simulink model "finalne_wo_simout"  (Simulink 7.3)
settings: Solver=ode45  StartTime=0.0  StopTime=1  RelTol=1e-3
libraries: powerlib x18
settings Model: Creator=me  LastModifiedBy=me

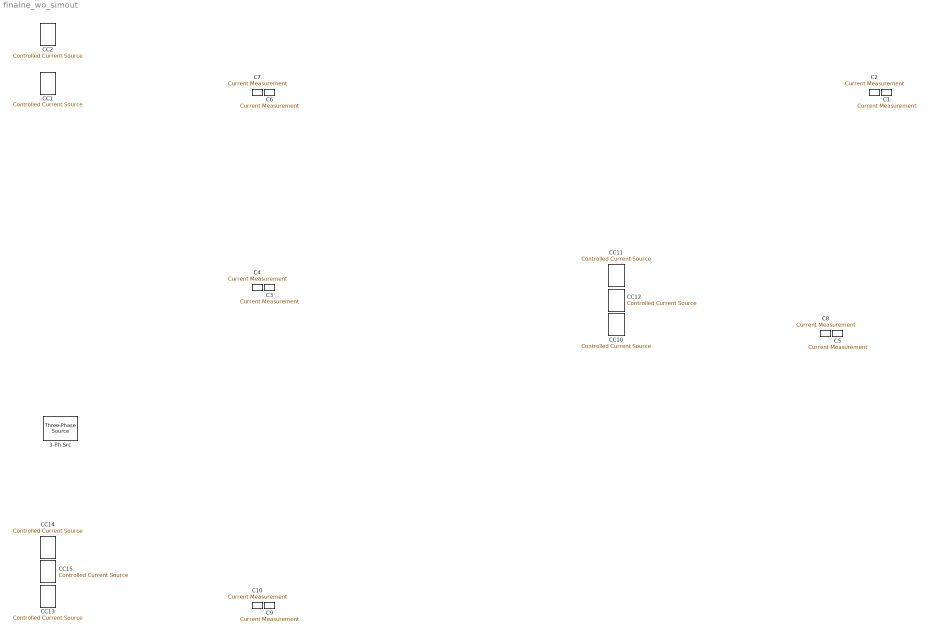
== system finalne_wo_simout ==
  3-Ph Src : powerlib/Electrical Sources/Three-Phase Source  DialogController=POWERSYS.PowerSysDialog  SystemSampleTime=-1  Voltage=380  PhaseAngle=0  Frequency=50  InternalConnection=Yn  SpecifyImpedance=on  Resistance=0.8929  Inductance=16.58e-3  ShortCircuitLevel=100e6  BaseVoltage=380  XRratio=7
  C{1..10} (10 alike) : powerlib/Measurements/Current Measurement  DialogController=POWERSYS.PowerSysDialog  SystemSampleTime=-1  PhasorSimulation=off  OutputType=Complex  PSBequivalent=0
  CC{1,10..15} (7 alike) : powerlib/Electrical Sources/Controlled Current Source  DialogController=POWERSYS.PowerSysDialog  SystemSampleTime=-1  Initialize=on  Source_Type=AC  Amplitude=0  Phase=0  Frequency=0  Measurements=None
  CC2 : Reference  SourceBlocK=powerlib/Electrkcal Wources/C/ntrolled CuRrent Source  SystemSampleTime=-1  Inherit="from model\""  Inherit=from model  Initialize="\u0000   on"  Amplitude=0  Phase=0  Frequency=0  Measurements=None
      settings: RTWMemSecFuncExecute="Inherit frgm model     RTWMemSecDataConstants"

== matlab function PF14 ==
  data: u input double; y output double
function y = fcn(u)
%#eml

y = cos(atan(u(2)/u(1)));

== matlab function PF15 ==
  data: u input double; y output double
function y = fcn(u)
%#eml

y = cos(atan(u(2)/u(1)));

== matlab function Subsystem1/1 constant power/Embedded MATLAB Function ==
  data: a input double; y output double
function y = fcn(a)
%#eml

y =[1/sqrt(3) 1/sqrt(3) 1/sqrt(3); sqrt(2)/sqrt(3) -sqrt(2)/(2*sqrt(3)) -sqrt(2)/(2*sqrt(3)); 0 1/sqrt(2) -1/sqrt(2)]*a;

== matlab function PF3 ==
  data: u input double; y output double
function y = fcn(u)
%#eml

y = cos(atan(u(2)/u(1)));

== matlab function Subsystem1/1 constant power/Embedded MATLAB Function1 ==
  data: b input double; y output double
function y = fcn(b)
%#eml

y = [1/sqrt(3) 1/sqrt(3) 1/sqrt(3); sqrt(2)/sqrt(3) -sqrt(2)/(2*sqrt(3)) -sqrt(2)/(2*sqrt(3)); 0 1/sqrt(2) -1/sqrt(2)]*b;

== matlab function PF8 ==
  data: u input double; y output double
function y = fcn(u)
%#eml

y = cos(atan(u(2)/u(1)));

== matlab function PF9 ==
  data: u input double; y output double
function y = fcn(u)
%#eml

y = cos(atan(u(2)/u(1)));

== matlab function Subsystem2/1 constant power/Embedded MATLAB Function ==
  data: a input double; y output double
function y = fcn(a)
%#eml

y =[1/sqrt(3) 1/sqrt(3) 1/sqrt(3); sqrt(2)/sqrt(3) -sqrt(2)/(2*sqrt(3)) -sqrt(2)/(2*sqrt(3)); 0 1/sqrt(2) -1/sqrt(2)]*a;

== matlab function Subsystem2/1 constant power/Embedded MATLAB Function1 ==
  data: b input double; y output double
function y = fcn(b)
%#eml

y = [1/sqrt(3) 1/sqrt(3) 1/sqrt(3); sqrt(2)/sqrt(3) -sqrt(2)/(2*sqrt(3)) -sqrt(2)/(2*sqrt(3)); 0 1/sqrt(2) -1/sqrt(2)]*b;

== matlab function Subsystem2/1 constant power/Embedded MATLAB Function3 ==
  data: h input double; y output double
function y = fcn(h)
%#eml

y =[1/sqrt(3) sqrt(2)/sqrt(3) 0 ;1/sqrt(3) -sqrt(2)/(2*sqrt(3)) 1/sqrt(2) ;1/sqrt(3) -sqrt(2)/(2*sqrt(3)) -1/sqrt(2)]*h;

== matlab function Subsystem2/1 constant power/Embedded MATLAB Function4 ==
  data: a input double; y output double
function y = fcn(a)
% #eml
if (a(2)^2+a(3)^2)==0
    y=[0; 0;0];
else
y =-[0;a(2);a(3)]*(a(4)/(a(2)^2+a(3)^2))+[a(5);a(6);a(7)];
end

== matlab function PF17 ==
  data: u input double; y output double
function y = fcn(u)
%#eml

y = cos(atan(u(2)/u(1)));

== matlab function PF18 ==
  data: u input double; y output double
function y = fcn(u)
%#eml

y = cos(atan(u(2)/u(1)));

== matlab function Subsystem2/2 unity PF/Embedded MATLAB Function ==
  data: a input double; y output double
function y = fcn(a)
%#eml

y =[1/sqrt(3) 1/sqrt(3) 1/sqrt(3); sqrt(2)/sqrt(3) -sqrt(2)/(2*sqrt(3)) -sqrt(2)/(2*sqrt(3)); 0 1/sqrt(2) -1/sqrt(2)]*a;

== matlab function Subsystem3/1 constant power/Embedded MATLAB Function ==
  data: a input double; y output double
function y = fcn(a)
%#eml

y =[1/sqrt(3) 1/sqrt(3) 1/sqrt(3); sqrt(2)/sqrt(3) -sqrt(2)/(2*sqrt(3)) -sqrt(2)/(2*sqrt(3)); 0 1/sqrt(2) -1/sqrt(2)]*a;

== matlab function Subsystem3/1 constant power/Embedded MATLAB Function1 ==
  data: b input double; y output double
function y = fcn(b)
%#eml

y = [1/sqrt(3) 1/sqrt(3) 1/sqrt(3); sqrt(2)/sqrt(3) -sqrt(2)/(2*sqrt(3)) -sqrt(2)/(2*sqrt(3)); 0 1/sqrt(2) -1/sqrt(2)]*b;

== matlab function PF11 ==
  data: u input double; y output double
function y = fcn(u)
%#eml

y = cos(atan(u(2)/u(1)));

== matlab function PF12 ==
  data: u input double; y output double
function y = fcn(u)
%#eml

y = cos(atan(u(2)/u(1)));

== matlab function Subsystem4/1 constant power/Embedded MATLAB Function ==
  data: a input double; y output double
function y = fcn(a)
%#eml

y =[1/sqrt(3) 1/sqrt(3) 1/sqrt(3); sqrt(2)/sqrt(3) -sqrt(2)/(2*sqrt(3)) -sqrt(2)/(2*sqrt(3)); 0 1/sqrt(2) -1/sqrt(2)]*a;

== matlab function Subsystem4/1 constant power/Embedded MATLAB Function1 ==
  data: b input double; y output double
function y = fcn(b)
%#eml

y = [1/sqrt(3) 1/sqrt(3) 1/sqrt(3); sqrt(2)/sqrt(3) -sqrt(2)/(2*sqrt(3)) -sqrt(2)/(2*sqrt(3)); 0 1/sqrt(2) -1/sqrt(2)]*b;

== matlab function Subsystem2/2 unity PF/Embedded MATLAB Function1 ==
  data: b input double; y output double
function y = fcn(b)
%#eml

y = [1/sqrt(3) 1/sqrt(3) 1/sqrt(3); sqrt(2)/sqrt(3) -sqrt(2)/(2*sqrt(3)) -sqrt(2)/(2*sqrt(3)); 0 1/sqrt(2) -1/sqrt(2)]*b;

== matlab function Subsystem/3 balanced currents /Embedded MATLAB Function ==
  data: u input double; iL_0dq output double
function iL_0dq = fcn(u)
%#eml

iL_0dq =[1/sqrt(3) 1/sqrt(3) 1/sqrt(3); sqrt(2)/sqrt(3) -sqrt(2)/(2*sqrt(3)) -sqrt(2)/(2*sqrt(3)); 0 1/sqrt(2) -1/sqrt(2)]*u;

== matlab function Subsystem2/2 unity PF/Embedded MATLAB Function2 ==
  data: a input double; y output double
function y = fcn(a)
% #eml

y =(a(1)^2+a(2)^2+a(3)^2);

== matlab function Subsystem2/2 unity PF/Embedded MATLAB Function3 ==
  data: h input double; y output double
function y = fcn(h)
%#eml

y =[1/sqrt(3) sqrt(2)/sqrt(3) 0 ;1/sqrt(3) -sqrt(2)/(2*sqrt(3)) 1/sqrt(2) ;1/sqrt(3) -sqrt(2)/(2*sqrt(3)) -1/sqrt(2)]*h;

== matlab function Subsystem2/2 unity PF/Embedded MATLAB Function4 ==
  data: a input double; y output double
function y = fcn(a)
% #eml
if a(7)<10
    y=[0; 0;0];
else
y =[a(1);a(2);a(3)]-[a(4);a(5);a(6)]*((a(8)/a(7)));
end

== matlab function Subsystem2/3 balanced currents /Embedded MATLAB Function ==
  data: u input double; iL_0dq output double
function iL_0dq = fcn(u)
%#eml

iL_0dq =[1/sqrt(3) 1/sqrt(3) 1/sqrt(3); sqrt(2)/sqrt(3) -sqrt(2)/(2*sqrt(3)) -sqrt(2)/(2*sqrt(3)); 0 1/sqrt(2) -1/sqrt(2)]*u;

== matlab function Subsystem2/3 balanced currents /Embedded MATLAB Function2 ==
  data: u input double; iL_0dq output double
function iL_0dq = fcn(u)
%#eml
if u(7)==0
    iL_0dq=[0;0;0];
else
iL_0dq =[u(1);u(2);u(3)]-(u(8)/u(7))*[0;u(5);u(6)];
end

== matlab function PF6 ==
  data: u input double; y output double
function y = fcn(u)
%#eml

y = cos(atan(u(2)/u(1)));

== matlab function Subsystem/3 balanced currents /Embedded MATLAB Function2 ==
  data: u input double; iL_0dq output double
function iL_0dq = fcn(u)
%#eml
if u(7)==0
    iL_0dq=[0;0;0];
else
iL_0dq =[u(1);u(2);u(3)]-(u(8)/u(7))*[0;u(5);u(6)];
end

== matlab function Subsystem/3 balanced currents /Embedded MATLAB Function3 ==
  data: u input double; y output double
function y = fcn(u)
%#eml

y =[1/sqrt(3) sqrt(2)/sqrt(3) 0 ;1/sqrt(3) -sqrt(2)/(2*sqrt(3)) 1/sqrt(2) ;1/sqrt(3) -sqrt(2)/(2*sqrt(3)) -1/sqrt(2)]*u;

== matlab function Subsystem/2 unity PF/Embedded MATLAB Function ==
  data: a input double; y output double
function y = fcn(a)
%#eml

y =[1/sqrt(3) 1/sqrt(3) 1/sqrt(3); sqrt(2)/sqrt(3) -sqrt(2)/(2*sqrt(3)) -sqrt(2)/(2*sqrt(3)); 0 1/sqrt(2) -1/sqrt(2)]*a;

== matlab function Subsystem/2 unity PF/Embedded MATLAB Function1 ==
  data: b input double; y output double
function y = fcn(b)
%#eml

y = [1/sqrt(3) 1/sqrt(3) 1/sqrt(3); sqrt(2)/sqrt(3) -sqrt(2)/(2*sqrt(3)) -sqrt(2)/(2*sqrt(3)); 0 1/sqrt(2) -1/sqrt(2)]*b;

== matlab function Subsystem/2 unity PF/Embedded MATLAB Function2 ==
  data: a input double; y output double
function y = fcn(a)
% #eml

y =(a(1)^2+a(2)^2+a(3)^2);

== matlab function Subsystem/2 unity PF/Embedded MATLAB Function3 ==
  data: h input double; y output double
function y = fcn(h)
%#eml

y =[1/sqrt(3) sqrt(2)/sqrt(3) 0 ;1/sqrt(3) -sqrt(2)/(2*sqrt(3)) 1/sqrt(2) ;1/sqrt(3) -sqrt(2)/(2*sqrt(3)) -1/sqrt(2)]*h;

== matlab function Subsystem/2 unity PF/Embedded MATLAB Function4 ==
  data: a input double; y output double
function y = fcn(a)
% #eml
if a(7)<10
    y=[0; 0;0];
else
y =[a(1);a(2);a(3)]-[a(4);a(5);a(6)]*((a(8)/a(7)));
end

== matlab function Subsystem/1 constant power/Embedded MATLAB Function ==
  data: a input double; y output double
function y = fcn(a)
%#eml

y =[1/sqrt(3) 1/sqrt(3) 1/sqrt(3); sqrt(2)/sqrt(3) -sqrt(2)/(2*sqrt(3)) -sqrt(2)/(2*sqrt(3)); 0 1/sqrt(2) -1/sqrt(2)]*a;

== matlab function Subsystem/1 constant power/Embedded MATLAB Function1 ==
  data: b input double; y output double
function y = fcn(b)
%#eml

y = [1/sqrt(3) 1/sqrt(3) 1/sqrt(3); sqrt(2)/sqrt(3) -sqrt(2)/(2*sqrt(3)) -sqrt(2)/(2*sqrt(3)); 0 1/sqrt(2) -1/sqrt(2)]*b;

== matlab function Subsystem/1 constant power/Embedded MATLAB Function3 ==
  data: h input double; y output double
function y = fcn(h)
%#eml

y =[1/sqrt(3) sqrt(2)/sqrt(3) 0 ;1/sqrt(3) -sqrt(2)/(2*sqrt(3)) 1/sqrt(2) ;1/sqrt(3) -sqrt(2)/(2*sqrt(3)) -1/sqrt(2)]*h;

== matlab function Subsystem/1 constant power/Embedded MATLAB Function4 ==
  data: a input double; y output double
function y = fcn(a)
% #eml
if (a(2)^2+a(3)^2)==0
    y=[0; 0;0];
else
y =-[0;a(2);a(3)]*(a(4)/(a(2)^2+a(3)^2))+[a(5);a(6);a(7)];
end

== matlab function Subsystem4/1 constant power/Embedded MATLAB Function3 ==
  data: h input double; y output double
function y = fcn(h)
%#eml

y =[1/sqrt(3) sqrt(2)/sqrt(3) 0 ;1/sqrt(3) -sqrt(2)/(2*sqrt(3)) 1/sqrt(2) ;1/sqrt(3) -sqrt(2)/(2*sqrt(3)) -1/sqrt(2)]*h;

== matlab function Subsystem4/1 constant power/Embedded MATLAB Function4 ==
  data: a input double; y output double
function y = fcn(a)
% #eml
if (a(2)^2+a(3)^2)==0
    y=[0; 0;0];
else
y =-[0;a(2);a(3)]*(a(4)/(a(2)^2+a(3)^2))+[a(5);a(6);a(7)];
end

== matlab function Subsystem4/2 unity PF/Embedded MATLAB Function ==
  data: a input double; y output double
function y = fcn(a)
%#eml

y =[1/sqrt(3) 1/sqrt(3) 1/sqrt(3); sqrt(2)/sqrt(3) -sqrt(2)/(2*sqrt(3)) -sqrt(2)/(2*sqrt(3)); 0 1/sqrt(2) -1/sqrt(2)]*a;

== matlab function Subsystem4/2 unity PF/Embedded MATLAB Function1 ==
  data: b input double; y output double
function y = fcn(b)
%#eml

y = [1/sqrt(3) 1/sqrt(3) 1/sqrt(3); sqrt(2)/sqrt(3) -sqrt(2)/(2*sqrt(3)) -sqrt(2)/(2*sqrt(3)); 0 1/sqrt(2) -1/sqrt(2)]*b;

== matlab function Subsystem4/2 unity PF/Embedded MATLAB Function2 ==
  data: a input double; y output double
function y = fcn(a)
% #eml

y =(a(1)^2+a(2)^2+a(3)^2);

== matlab function Subsystem4/2 unity PF/Embedded MATLAB Function3 ==
  data: h input double; y output double
function y = fcn(h)
%#eml

y =[1/sqrt(3) sqrt(2)/sqrt(3) 0 ;1/sqrt(3) -sqrt(2)/(2*sqrt(3)) 1/sqrt(2) ;1/sqrt(3) -sqrt(2)/(2*sqrt(3)) -1/sqrt(2)]*h;

== matlab function Subsystem4/2 unity PF/Embedded MATLAB Function4 ==
  data: a input double; y output double
function y = fcn(a)
% #eml
if a(7)<10
    y=[0; 0;0];
else
y =[a(1);a(2);a(3)]-[a(4);a(5);a(6)]*((a(8)/a(7)));
end

== matlab function Subsystem4/3 balanced currents /Embedded MATLAB Function ==
  data: u input double; iL_0dq output double
function iL_0dq = fcn(u)
%#eml

iL_0dq =[1/sqrt(3) 1/sqrt(3) 1/sqrt(3); sqrt(2)/sqrt(3) -sqrt(2)/(2*sqrt(3)) -sqrt(2)/(2*sqrt(3)); 0 1/sqrt(2) -1/sqrt(2)]*u;

== matlab function Subsystem4/3 balanced currents /Embedded MATLAB Function2 ==
  data: u input double; iL_0dq output double
function iL_0dq = fcn(u)
%#eml
if u(7)==0
    iL_0dq=[0;0;0];
else
iL_0dq =[u(1);u(2);u(3)]-(u(8)/u(7))*[0;u(5);u(6)];
end

== matlab function Subsystem3/1 constant power/Embedded MATLAB Function3 ==
  data: h input double; y output double
function y = fcn(h)
%#eml

y =[1/sqrt(3) sqrt(2)/sqrt(3) 0 ;1/sqrt(3) -sqrt(2)/(2*sqrt(3)) 1/sqrt(2) ;1/sqrt(3) -sqrt(2)/(2*sqrt(3)) -1/sqrt(2)]*h;

== matlab function Subsystem3/1 constant power/Embedded MATLAB Function4 ==
  data: a input double; y output double
function y = fcn(a)
% #eml
if (a(2)^2+a(3)^2)==0
    y=[0; 0;0];
else
y =-[0;a(2);a(3)]*(a(4)/(a(2)^2+a(3)^2))+[a(5);a(6);a(7)];
end

== matlab function Subsystem3/2 unity PF/Embedded MATLAB Function ==
  data: a input double; y output double
function y = fcn(a)
%#eml

y =[1/sqrt(3) 1/sqrt(3) 1/sqrt(3); sqrt(2)/sqrt(3) -sqrt(2)/(2*sqrt(3)) -sqrt(2)/(2*sqrt(3)); 0 1/sqrt(2) -1/sqrt(2)]*a;

== matlab function Subsystem3/2 unity PF/Embedded MATLAB Function1 ==
  data: b input double; y output double
function y = fcn(b)
%#eml

y = [1/sqrt(3) 1/sqrt(3) 1/sqrt(3); sqrt(2)/sqrt(3) -sqrt(2)/(2*sqrt(3)) -sqrt(2)/(2*sqrt(3)); 0 1/sqrt(2) -1/sqrt(2)]*b;

== matlab function Subsystem3/2 unity PF/Embedded MATLAB Function2 ==
  data: a input double; y output double
function y = fcn(a)
% #eml

y =(a(1)^2+a(2)^2+a(3)^2);

== matlab function Subsystem3/2 unity PF/Embedded MATLAB Function3 ==
  data: h input double; y output double
function y = fcn(h)
%#eml

y =[1/sqrt(3) sqrt(2)/sqrt(3) 0 ;1/sqrt(3) -sqrt(2)/(2*sqrt(3)) 1/sqrt(2) ;1/sqrt(3) -sqrt(2)/(2*sqrt(3)) -1/sqrt(2)]*h;

== matlab function Subsystem3/2 unity PF/Embedded MATLAB Function4 ==
  data: a input double; y output double
function y = fcn(a)
% #eml
if a(7)<10
    y=[0; 0;0];
else
y =[a(1);a(2);a(3)]-[a(4);a(5);a(6)]*((a(8)/a(7)));
end

== matlab function Subsystem3/3 balanced currents /Embedded MATLAB Function ==
  data: u input double; iL_0dq output double
function iL_0dq = fcn(u)
%#eml

iL_0dq =[1/sqrt(3) 1/sqrt(3) 1/sqrt(3); sqrt(2)/sqrt(3) -sqrt(2)/(2*sqrt(3)) -sqrt(2)/(2*sqrt(3)); 0 1/sqrt(2) -1/sqrt(2)]*u;

== matlab function Subsystem3/3 balanced currents /Embedded MATLAB Function2 ==
  data: u input double; iL_0dq output double
function iL_0dq = fcn(u)
%#eml
if u(7)==0
    iL_0dq=[0;0;0];
else
iL_0dq =[u(1);u(2);u(3)]-(u(8)/u(7))*[0;u(5);u(6)];
end

== matlab function Subsystem1/1 constant power/Embedded MATLAB Function3 ==
  data: h input double; y output double
function y = fcn(h)
%#eml

y =[1/sqrt(3) sqrt(2)/sqrt(3) 0 ;1/sqrt(3) -sqrt(2)/(2*sqrt(3)) 1/sqrt(2) ;1/sqrt(3) -sqrt(2)/(2*sqrt(3)) -1/sqrt(2)]*h;

== matlab function Subsystem1/1 constant power/Embedded MATLAB Function4 ==
  data: a input double; y output double
function y = fcn(a)
% #eml
if (a(2)^2+a(3)^2)==0
    y=[0; 0;0];
else
y =-[0;a(2);a(3)]*(a(4)/(a(2)^2+a(3)^2))+[a(5);a(6);a(7)];
end

== matlab function Subsystem1/2 unity PF/Embedded MATLAB Function ==
  data: a input double; y output double
function y = fcn(a)
%#eml

y =[1/sqrt(3) 1/sqrt(3) 1/sqrt(3); sqrt(2)/sqrt(3) -sqrt(2)/(2*sqrt(3)) -sqrt(2)/(2*sqrt(3)); 0 1/sqrt(2) -1/sqrt(2)]*a;

== matlab function Subsystem1/2 unity PF/Embedded MATLAB Function1 ==
  data: b input double; y output double
function y = fcn(b)
%#eml

y = [1/sqrt(3) 1/sqrt(3) 1/sqrt(3); sqrt(2)/sqrt(3) -sqrt(2)/(2*sqrt(3)) -sqrt(2)/(2*sqrt(3)); 0 1/sqrt(2) -1/sqrt(2)]*b;

== matlab function Subsystem1/2 unity PF/Embedded MATLAB Function2 ==
  data: a input double; y output double
function y = fcn(a)
% #eml

y =(a(1)^2+a(2)^2+a(3)^2);

== matlab function Subsystem1/2 unity PF/Embedded MATLAB Function3 ==
  data: h input double; y output double
function y = fcn(h)
%#eml

y =[1/sqrt(3) sqrt(2)/sqrt(3) 0 ;1/sqrt(3) -sqrt(2)/(2*sqrt(3)) 1/sqrt(2) ;1/sqrt(3) -sqrt(2)/(2*sqrt(3)) -1/sqrt(2)]*h;

== matlab function Subsystem1/2 unity PF/Embedded MATLAB Function4 ==
  data: a input double; y output double
function y = fcn(a)
% #eml
if a(7)<10
    y=[0; 0;0];
else
y =[a(1);a(2);a(3)]-[a(4);a(5);a(6)]*((a(8)/a(7)));
end

== matlab function Subsystem1/3 balanced currents /Embedded MATLAB Function ==
  data: u input double; iL_0dq output double
function iL_0dq = fcn(u)
%#eml

iL_0dq =[1/sqrt(3) 1/sqrt(3) 1/sqrt(3); sqrt(2)/sqrt(3) -sqrt(2)/(2*sqrt(3)) -sqrt(2)/(2*sqrt(3)); 0 1/sqrt(2) -1/sqrt(2)]*u;

== matlab function Subsystem1/3 balanced currents /Embedded MATLAB Function2 ==
  data: u input double; iL_0dq output double
function iL_0dq = fcn(u)
%#eml
if u(7)==0
    iL_0dq=[0;0;0];
else
iL_0dq =[u(1);u(2);u(3)]-(u(8)/u(7))*[0;u(5);u(6)];
end

== matlab function Subsystem2/3 balanced currents /Embedded MATLAB Function3 ==
  data: u input double; y output double
function y = fcn(u)
%#eml

y =[1/sqrt(3) sqrt(2)/sqrt(3) 0 ;1/sqrt(3) -sqrt(2)/(2*sqrt(3)) 1/sqrt(2) ;1/sqrt(3) -sqrt(2)/(2*sqrt(3)) -1/sqrt(2)]*u;

== matlab function Subsystem4/3 balanced currents /Embedded MATLAB Function3 ==
  data: u input double; y output double
function y = fcn(u)
%#eml

y =[1/sqrt(3) sqrt(2)/sqrt(3) 0 ;1/sqrt(3) -sqrt(2)/(2*sqrt(3)) 1/sqrt(2) ;1/sqrt(3) -sqrt(2)/(2*sqrt(3)) -1/sqrt(2)]*u;

== matlab function Subsystem1/3 balanced currents /Embedded MATLAB Function3 ==
  data: u input double; y output double
function y = fcn(u)
%#eml

y =[1/sqrt(3) sqrt(2)/sqrt(3) 0 ;1/sqrt(3) -sqrt(2)/(2*sqrt(3)) 1/sqrt(2) ;1/sqrt(3) -sqrt(2)/(2*sqrt(3)) -1/sqrt(2)]*u;

== matlab function Subsystem3/3 balanced currents /Embedded MATLAB Function3 ==
  data: u input double; y output double
function y = fcn(u)
%#eml

y =[1/sqrt(3) sqrt(2)/sqrt(3) 0 ;1/sqrt(3) -sqrt(2)/(2*sqrt(3)) 1/sqrt(2) ;1/sqrt(3) -sqrt(2)/(2*sqrt(3)) -1/sqrt(2)]*u;
